simulink model "sampleModel1520"  (R2023a)
settings: Solver=VariableStepAuto  StartTime=0.0  StopTime=10.0  RelTol=1e-3
libraries: simulink x5, hdlsllib x5
settings Model: Creator=user1  LastModifiedBy=user1

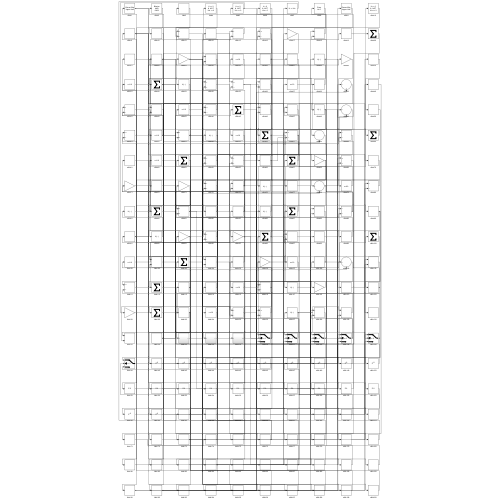
[thumbnail: Simulink's stored preview of the top-level diagram]
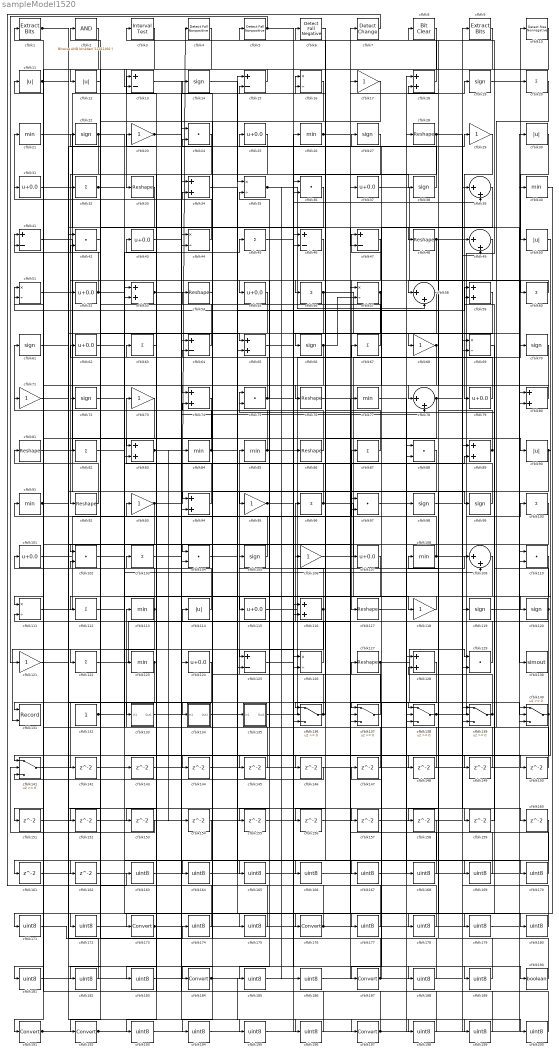
== system sampleModel1520 ==
  cfblk1 : simulink/Logic and Bit Operations/Extract Bits  bitsToExtract=Upper half  numBits=8  bitIdxRange=[0 7]  outScalingMode=Preserve fixed-point scaling
      settings: LibrarySourceBlock=|
      | hdlsllib/Logic and Bit
      | Operations/Extract Bits
  cfblk10 : hdlsllib/Logic and Bit Operations/Detect Rise Nonnegative  vinit=0  OutDataTypeStr=boolean
  cfblk{20,32,45,56,60,63,67,82,87,96,100,103,112,122} (14 alike) : Sum  Inputs=+
  cfblk{25,31,37,43,52,55,62,79,101,107,115,124} (12 alike) : Bias  Bias=0.0  SaturateOnIntegerOverflow=off
  cfblk{24,36,42,75,88,97,102,104,110,129} (10 alike) : DotProduct  OutDataTypeStr=Inherit: Inherit via internal rule
  cfblk{14,19,22,27,38,61,66,70,72,98..99,105,119..120} (14 alike) : Signum
  cfblk{17,23,29,68,71,73,93,95,106,118,121} (11 alike) : Gain
  cfblk{21,26,40,77,84..85,91,108,113,123} (10 alike) : MinMax
  cfblk{39,49,58,78,109} (5 alike) : Sum  Inputs=|++
  cfblk{11..12,30,50,90,114} (6 alike) : Abs  SaturateOnIntegerOverflow=off
  cfblk{16,35,44,51,57,69,111,126} (8 alike) : Product  Inputs=*/  RndMeth=Zero  SaturateOnIntegerOverflow=on
  cfblk{18,34,53,59,65,74,80,83,89,94,116,128} (12 alike) : Sum
  cfblk{28,33,48,54,76,81,86,92,117,127} (10 alike) : Reshape
  cfblk{13,15,41,46..47,64,125} (7 alike) : Sum  Inputs=+-
  cfblk130 : ToWorkspace  VariableName=simout  SaveFormat=Timeseries  SampleTime=-1
  cfblk131 : Record  FileSettingsInternal="{\"entries\":[{\"content\":{\"excelSettings\":{\"content\":{},\"type\":\"Streamout.ExcelSettings\"}},\"type\":\"Streamout.FileSettingStorage\",\"uuid\":\"\"}],\"packageUris\":[\"http:\\/\\/schema.mathworks.com\\/mf0\\/streamout_blocks\\/R2020a\"],\"version\":\"1.0\"}"  Layout=[1 1]  SignalsInternal="{\"entries\":[{\"content\":{\"signals\":[{\"content\":{\"blockPath\":[],\"dimensions\":[1],\"domain\":\"\",\"lineColor\":\"#a2142f\",\"plots\":[1],\"port\":1,\"signalID\":1453,\"signalName\":\"XY Graph:1\"},\"type\":\"RecordBlkView.Signal\",\"uuid\":\"\"},{\"content\":{\"blockPath\":[],\"dimensions\":[1],\"domain\":\"\",\"lineColor\":\"#139fff\",\"plots\":[1],\"port\":2,\"signalID\":1456,\"signalName\":\"XY Graph:2\"},\"type\":\"RecordBlkView.Signal\",\"uuid\":\"\"}]},\"type\":\"RecordBlkView.InputSignals\",\"uuid\":\"\"}],\"packageUris\":[\"http:\\/\\/schema.mathworks.com\\/mf0\\/streamout_blocks\\/R2020a\"],\"version\":\"1.0\"}"  VisualizationBindings="{\"xyplotplugin\":{\"info\":[{\"series\":[{\"bindingParametersList\":[{\"parameter\":\"X-Axis\",\"signalID\":1453,\"signalName\":\"XY Graph:1\"},{\"parameter\":\"Y-Axis\",\"signalID\":1456,\"signalName\":\"XY Graph:2\"}],\"seriesID\":12025}],\"subplotID\":1}]}}"  CompatibilityTag=XY  st=-1
  cfblk132 : Constant  SampleTime=-1
  cfblk133 : Subsystem
      settings: LibrarySourceBlock=|
      | hdlsllib/Ports &
      | Subsystems/Subsystem
  cfblk134 : Subsystem
      settings: LibrarySourceBlock=|
      | hdlsllib/Ports &
      | Subsystems/Subsystem
  cfblk135 : Subsystem
      settings: LibrarySourceBlock=|
      | hdlsllib/Ports &
      | Subsystems/Subsystem
  cfblk{136..141} (6 alike) : Switch  SaturateOnIntegerOverflow=off  InputSameDT=off
  cfblk{142..162} (21 alike) : Delay  SampleTime=1
  cfblk{163..172,174..175,177..183,185..186,188..189,193..196,198..200} (30 alike) : DataTypeConversion  OutDataTypeStr=uint8  SaturateOnIntegerOverflow=off  RndMeth=Floor
  cfblk{173,176,184,187,191..192,197} (7 alike) : DataTypeConversion  SaturateOnIntegerOverflow=off  RndMeth=Floor
  cfblk190 : DataTypeConversion  OutDataTypeStr=boolean  SaturateOnIntegerOverflow=off  RndMeth=Floor
  cfblk2 : simulink/Logic and Bit Operations/Bitwise Operator  logicop=AND  UseBitMask=on  BitMask=bin2dec('11011001')  BitMaskRealWorld=Stored Integer
      settings: LibrarySourceBlock=|
      | hdlsllib/Logic and Bit
      | Operations/Bitwise
      | Operator
  cfblk3 : hdlsllib/Logic and Bit Operations/Interval Test  IntervalClosedRight=on  uplimit=0.5  IntervalClosedLeft=on  lowlimit=-0.5  OutDataTypeStr=boolean
  cfblk4 : hdlsllib/Logic and Bit Operations/Detect Fall Nonpositive  vinit=0  OutDataTypeStr=boolean
  cfblk5 : hdlsllib/Logic and Bit Operations/Detect Fall Nonpositive  vinit=0  OutDataTypeStr=boolean
  cfblk6 : hdlsllib/Logic and Bit Operations/Detect Fall Negative  vinit=0  OutDataTypeStr=boolean
  cfblk7 : simulink/Logic and Bit Operations/Detect Change  vinit=0  OutDataTypeStr=boolean
      settings: LibrarySourceBlock=|
      | hdlsllib/Logic and Bit
      | Operations/Detect
      | Change
  cfblk8 : simulink/Logic and Bit Operations/Bit Clear  iBit=0
      settings: LibrarySourceBlock=|
      | hdlsllib/Logic and Bit
      | Operations/Bit Clear
  cfblk9 : simulink/Logic and Bit Operations/Extract Bits  bitsToExtract=Upper half  numBits=8  bitIdxRange=[0 7]  outScalingMode=Preserve fixed-point scaling
      settings: LibrarySourceBlock=|
      | hdlsllib/Logic and Bit
      | Operations/Extract Bits
  wires:
  cfblk25/1 -> cfblk92/1
  cfblk47/1 -> cfblk117/1
  cfblk48/1 -> cfblk58/1, cfblk104/2, cfblk78/1, cfblk49/2
  cfblk116/1 -> cfblk85/1, cfblk185/1
  cfblk135/1(Out1) -> cfblk67/1
  cfblk138/1 -> cfblk3/1, cfblk18/2
  cfblk93/1 -> cfblk4/1, cfblk152/1
  cfblk3/1 -> cfblk33/1
  cfblk20/1 -> cfblk113/1
  cfblk113/1 -> cfblk101/1, cfblk131/2
  cfblk106/1 -> cfblk10/1
  cfblk99/1 -> cfblk23/1
  cfblk29/1 -> cfblk79/1
  cfblk126/1 -> cfblk96/1
  cfblk105/1 -> cfblk91/1
  cfblk127/1 -> cfblk129/1, cfblk140/2, cfblk137/2
  cfblk24/1 -> cfblk173/1
  cfblk108/1 -> cfblk100/1, cfblk31/1
  cfblk51/1 -> cfblk84/1
  cfblk101/1 -> cfblk15/1
  cfblk56/1 -> cfblk130/1, cfblk155/1
  cfblk94/1 -> cfblk73/1
  cfblk122/1 -> cfblk37/1
  cfblk57/1 -> cfblk74/1, cfblk194/1
  cfblk41/1 -> cfblk94/1
  cfblk37/1 -> cfblk119/1
  cfblk115/1 -> cfblk109/1
  cfblk91/1 -> cfblk99/1, cfblk107/1
  cfblk84/1 -> cfblk61/1, cfblk59/1
  cfblk129/1 -> cfblk27/1
  cfblk120/1 -> cfblk75/1, cfblk111/2
  cfblk88/1 -> cfblk184/1
  cfblk30/1 -> cfblk50/1
  cfblk128/1 -> cfblk187/1
  cfblk19/1 -> cfblk20/1
  cfblk111/1 -> cfblk87/1
  cfblk81/1 -> cfblk15/2
  cfblk38/1 -> cfblk25/1
  cfblk5/1 -> cfblk121/1, cfblk38/1
  cfblk89/1 -> cfblk62/1, cfblk51/1
  cfblk21/1 -> cfblk70/1
  cfblk79/1 -> cfblk47/1
  cfblk103/1 -> cfblk197/1
  cfblk90/1 -> cfblk141/1, cfblk178/1
  cfblk22/1 -> cfblk134/1(In1), cfblk90/1, cfblk32/1
  cfblk14/1 -> cfblk35/1
  cfblk70/1 -> cfblk83/1
  cfblk83/1 -> cfblk126/2, cfblk154/1
  cfblk15/1 -> cfblk12/1
  cfblk74/1 -> cfblk83/2
  cfblk139/1 -> cfblk8/1, cfblk108/1
  cfblk66/1 -> cfblk94/2, cfblk57/2
  cfblk134/1(Out1) -> cfblk135/1(In1)
  cfblk27/1 -> cfblk122/1
  cfblk59/1 -> cfblk66/1
  cfblk119/1 -> cfblk80/1
  cfblk60/1 -> cfblk55/1
  cfblk92/1 -> cfblk81/1
  cfblk31/1 -> cfblk123/1
  cfblk8/1 -> cfblk116/2
  cfblk52/1 -> cfblk45/1, cfblk41/1, cfblk177/1
  cfblk26/1 -> cfblk19/1, cfblk156/1
  cfblk137/1 -> cfblk105/1
  cfblk65/1 -> cfblk68/1
  cfblk140/1 -> cfblk74/2, cfblk153/1
  cfblk136/1 -> cfblk114/1, cfblk16/2, cfblk106/1
  cfblk39/1 -> cfblk77/1
  cfblk96/1 -> cfblk13/1, cfblk138/2
  cfblk112/1 -> cfblk118/1
  cfblk42/1 -> cfblk82/1
  cfblk107/1 -> cfblk112/1
  cfblk62/1 -> cfblk125/1
  cfblk123/1 -> cfblk133/1(In1), cfblk161/1
  cfblk87/1 -> cfblk6/1
  cfblk35/1 -> cfblk58/2, cfblk136/2
  cfblk33/1 -> cfblk72/1
  cfblk133/1(Out1) -> cfblk138/1
  cfblk2/1 -> cfblk191/1
  cfblk10/1 -> cfblk102/1
  cfblk9/1 -> cfblk56/1
  cfblk28/1 -> cfblk36/2, cfblk60/1
  cfblk4/1 -> cfblk13/2
  cfblk11/1 -> cfblk48/1, cfblk137/1, cfblk159/1
  cfblk46/1 -> cfblk192/1
  cfblk132/1 -> cfblk109/2, cfblk89/2
  cfblk53/1 -> cfblk16/1, cfblk196/1
  cfblk44/1 -> cfblk21/1
  cfblk75/1 -> cfblk64/2, cfblk35/2, cfblk189/1
  cfblk78/1 -> cfblk9/1, cfblk136/1
  cfblk80/1 -> cfblk76/1
  cfblk102/1 -> cfblk53/2
  cfblk23/1 -> cfblk125/2, cfblk78/2, cfblk157/1
  cfblk50/1 -> cfblk120/1
  cfblk114/1 -> cfblk42/2
  cfblk64/1 -> cfblk22/1
  cfblk18/1 -> cfblk5/1
  cfblk100/1 -> cfblk131/1
  cfblk54/1 -> cfblk104/1
  cfblk85/1 -> cfblk126/1, cfblk41/2, cfblk51/2
  cfblk32/1 -> cfblk44/2, cfblk138/3
  cfblk95/1 -> cfblk39/2, cfblk186/1
  cfblk118/1 -> cfblk115/1
  cfblk1/1 -> cfblk65/1, cfblk47/2
  cfblk141/1 -> cfblk28/1
  cfblk121/1 -> cfblk29/1
  cfblk67/1 -> cfblk14/1
  cfblk68/1 -> cfblk95/1, cfblk111/1
  cfblk86/1 -> cfblk11/1
  cfblk12/1 -> cfblk52/1
  cfblk34/1 -> cfblk176/1
  cfblk124/1 -> cfblk142/1
  cfblk142/1 -> cfblk129/2
  cfblk82/1 -> cfblk143/1
  cfblk143/1 -> cfblk80/2
  cfblk16/1 -> cfblk144/1
  cfblk144/1 -> cfblk39/1
  cfblk49/1 -> cfblk145/1
  cfblk145/1 -> cfblk53/1
  cfblk104/1 -> cfblk146/1
  cfblk146/1 -> cfblk141/3
  cfblk147/1 -> cfblk75/2
  cfblk72/1 -> cfblk148/1
  cfblk148/1 -> cfblk36/1
  cfblk117/1 -> cfblk149/1
  cfblk149/1 -> cfblk116/1
  cfblk45/1 -> cfblk150/1
  cfblk150/1 -> cfblk1/1
  cfblk73/1 -> cfblk151/1
  cfblk151/1 -> cfblk18/1
  cfblk153/1 -> cfblk141/2
  cfblk155/1 -> cfblk139/3
  cfblk156/1 -> cfblk137/3
  cfblk157/1 -> cfblk139/2
  cfblk109/1 -> cfblk158/1
  cfblk159/1 -> cfblk59/2
  cfblk98/1 -> cfblk160/1
  cfblk161/1 -> cfblk65/2
  cfblk55/1 -> cfblk162/1
  cfblk162/1 -> cfblk64/1
  cfblk7/1 -> cfblk163/1
  cfblk163/1 -> cfblk124/1
  cfblk58/1 -> cfblk164/1
  cfblk164/1 -> cfblk7/1
  cfblk110/1 -> cfblk165/1
  cfblk165/1 -> cfblk26/1
  cfblk6/1 -> cfblk166/1
  cfblk166/1 -> cfblk110/1
  cfblk125/1 -> cfblk167/1
  cfblk167/1 -> cfblk110/2
  cfblk97/1 -> cfblk168/1
  cfblk168/1 -> cfblk127/1
  cfblk77/1 -> cfblk169/1
  cfblk169/1 -> cfblk97/1
  cfblk152/1 -> cfblk170/1
  cfblk170/1 -> cfblk97/2
  cfblk40/1 -> cfblk171/1
  cfblk36/1 -> cfblk172/1
  cfblk172/1 -> cfblk40/1
  cfblk173/1 -> cfblk89/1, cfblk198/1
  cfblk171/1 -> cfblk174/1
  cfblk174/1 -> cfblk24/1
  cfblk158/1 -> cfblk175/1
  cfblk175/1 -> cfblk24/2
  cfblk176/1 -> cfblk102/2, cfblk93/1
  cfblk177/1 -> cfblk34/1
  cfblk178/1 -> cfblk34/2
  cfblk69/1 -> cfblk179/1
  cfblk179/1 -> cfblk30/1
  cfblk76/1 -> cfblk180/1
  cfblk180/1 -> cfblk69/1
  cfblk154/1 -> cfblk181/1
  cfblk181/1 -> cfblk69/2
  cfblk17/1 -> cfblk182/1
  cfblk182/1 -> cfblk42/1
  cfblk63/1 -> cfblk183/1
  cfblk183/1 -> cfblk17/1
  cfblk184/1 -> cfblk57/1, cfblk200/1
  cfblk185/1 -> cfblk88/1
  cfblk186/1 -> cfblk88/2
  cfblk187/1 -> cfblk147/1, cfblk54/1
  cfblk13/1 -> cfblk188/1
  cfblk188/1 -> cfblk128/1
  cfblk189/1 -> cfblk128/2
  cfblk61/1 -> cfblk190/1
  cfblk190/1 -> cfblk2/1
  cfblk191/1 -> cfblk140/3, cfblk140/1
  cfblk192/1 -> cfblk136/3, cfblk98/1, cfblk86/1
  cfblk160/1 -> cfblk193/1
  cfblk193/1 -> cfblk46/1
  cfblk194/1 -> cfblk46/2
  cfblk43/1 -> cfblk195/1
  cfblk195/1 -> cfblk49/1
  cfblk196/1 -> cfblk43/1
  cfblk197/1 -> cfblk139/1, cfblk63/1
  cfblk198/1 -> cfblk103/1
  cfblk71/1 -> cfblk199/1
  cfblk199/1 -> cfblk44/1
  cfblk200/1 -> cfblk71/1

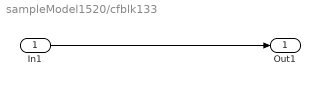
== system sampleModel1520/cfblk133 ==
  In1 : Inport
  Out1 : Outport
  wires:
  In1/1 -> Out1/1

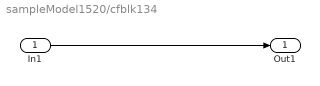
== system sampleModel1520/cfblk134 ==
  In1 : Inport
  Out1 : Outport
  wires:
  In1/1 -> Out1/1

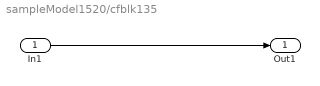
== system sampleModel1520/cfblk135 ==
  In1 : Inport
  Out1 : Outport
  wires:
  In1/1 -> Out1/1
